simulink model "cochons_nofail"  (R2014b)
settings: Solver=ode45  StartTime=0.0  StopTime=12000  RelTol=1e-3
libraries: simulink x2
settings Model: TunableVars=p  TunableVarsStorageClass=Auto  Creator=ltraonou  LastModifiedBy=ltraonou
settings SolverCC: ShapePreserveControl=EnableAll
settings DataIOCC: FinalStateName=last_state  InitialState=last_state  LimitDataPoints=off  SaveFormat=StructureWithTime  SaveOutput=off  SaveTime=off
settings OptimizationCC: InlineParams=on
settings DebuggingCC: UnderspecifiedInitializationDetection=Classic  MergeDetectMultiDrivingBlocksExec=none  MultiTaskDSMMsg=warning  MultiTaskCondExecSysMsg=none
settings RTWCC: IncludeERTFirstTime=on

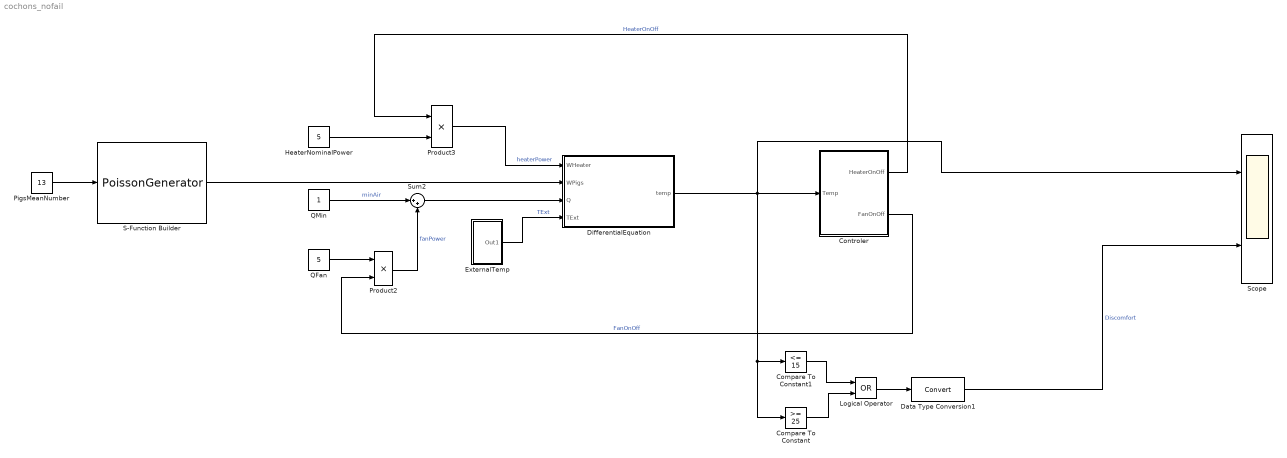
== system cochons_nofail ==
  Compare To Constant : simulink/Logic and Bit Operations/Compare To Constant  relop=>=  const=25  OutDataTypeStr=boolean
  Compare To Constant1 : simulink/Logic and Bit Operations/Compare To Constant  relop=<=  const=15  OutDataTypeStr=boolean
  Controler : Subsystem
  Data Type Conversion1 : DataTypeConversion
  DifferentialEquation : Subsystem
  ExternalTemp : Subsystem
  HeaterNominalPower : Constant  Value=5
  Logical Operator : Logic  Operator=OR  AllPortsSameDT=off  OutDataTypeStr=boolean
  PigsMeanNumber : Constant  Value=13
  Product2 : Product
  Product3 : Product
  QFan : Constant  Value=5
  QMin : Constant
  S-Function Builder : S-Function  InitFcn=try, set_param(gcb,'FunctionName','PoissonGenerator'), end  FunctionName=PoissonGenerator  SFunctionModules=PoissonGenerator_wrapper  EnableBusSupport=off  mask(S-Function Builder){}
      mask help: Simulink:masks:SFunctionBuilder_MD
      mask init:
      | val = [[.9  0.75 0.75 1 1 .9 .9 1]',[1 1 0.75 0.75 .9 .9 1 .9]'];try , sys = get_param(gcb,'SfunBuilderFcnName');if isempty(sys), sys = get_param(gcb,'FunctionName'); end,catch, sys = get_param(gcb,'FunctionName'); end
      settings: CopyFcn=set_param(gcbh,'LinkStatus','none')  PreSaveFcn=try, set_param(gcb,'FunctionName','PoissonGenerator'), end  OpenFcn=sfunctionwizard(gcbh)
      mask Display: plot(val(:,1),val(:,2)),disp(sys), port_label('input',1,'lambda'), port_label('output',1,'y')
  Scope : Scope  NumInputPorts=2
      settings: TimeRange=200000  YMin=-5~-5  YMax=5~5
  Sum2 : Sum  Inputs=|++
  wires:
  QFan/1 -> Product2/1
  QMin/1 -> Sum2/1  "minAir"
  Product2/1 -> Sum2/2  "fanPower"
  Product3/1 -> DifferentialEquation/1(WHeater)  "heaterPower"
  HeaterNominalPower/1 -> Product3/2
  Controler/2(FanOnOff) -> Product2/2  "FanOnOff"
  Controler/1(HeaterOnOff) -> Product3/1  "HeaterOnOff"
  Data Type Conversion1/1 -> Scope/2  "Discomfort"
  DifferentialEquation/1(temp) -> Controler/1(Temp), Scope/1, Compare To Constant/1, Compare To Constant1/1
  S-Function Builder/1 -> DifferentialEquation/2(WPigs)
  Sum2/1 -> DifferentialEquation/3(Q)
  PigsMeanNumber/1 -> S-Function Builder/1
  ExternalTemp/1(Out1) -> DifferentialEquation/4(TExt)  "TExt"
  Compare To Constant1/1 -> Logical Operator/1
  Compare To Constant/1 -> Logical Operator/2
  Logical Operator/1 -> Data Type Conversion1/1

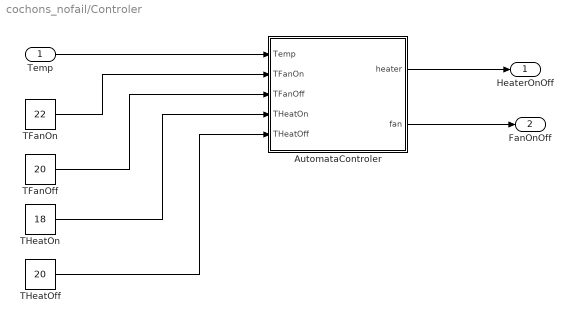
== system cochons_nofail/Controler ==
  Temp : Inport
  AutomataControler : Stateflow chart  TreatAsAtomicUnit=on
  TFanOff : Constant  Value=20
  TFanOn : Constant  Value=22
  THeatOff : Constant  Value=20
  THeatOn : Constant  Value=18
  HeaterOnOff : Outport
  FanOnOff : Outport  Port=2
  wires:
  Temp/1 -> AutomataControler/1(Temp)
  TFanOn/1 -> AutomataControler/2(TFanOn)
  THeatOn/1 -> AutomataControler/4(THeatOn)
  THeatOff/1 -> AutomataControler/5(THeatOff)
  TFanOff/1 -> AutomataControler/3(TFanOff)
  AutomataControler/2(fan) -> FanOnOff/1
  AutomataControler/1(heater) -> HeaterOnOff/1

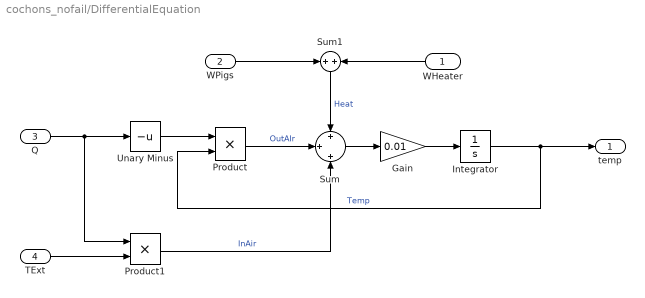
== system cochons_nofail/DifferentialEquation ==
  WHeater : Inport
  WPigs : Inport  Port=2
  Q : Inport  Port=3
  TExt : Inport  Port=4
  Gain : Gain  Gain=0.01
  Integrator : Integrator  InitialCondition=20
  Product : Product
  Product1 : Product
  Sum : Sum  Inputs=+|+|+
  Sum1 : Sum  Inputs=+|+
  Unary Minus : UnaryMinus
  temp : Outport
  wires:
  WHeater/1 -> Sum1/2
  Sum1/1 -> Sum/1  "Heat"
  Unary Minus/1 -> Product/1
  Product1/1 -> Sum/3  "InAir"
  Product/1 -> Sum/2  "OutAIr"
  Q/1 -> Product1/1, Unary Minus/1
  Sum/1 -> Gain/1
  Gain/1 -> Integrator/1
  WPigs/1 -> Sum1/1
  Integrator/1 -> Product/2, temp/1  "Temp"
  TExt/1 -> Product1/2

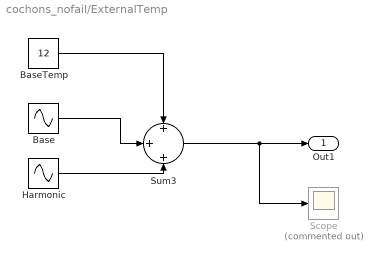
== system cochons_nofail/ExternalTemp ==
  Base : Sin  Amplitude=10  Frequency=0.01  SampleTime=0
  BaseTemp : Constant  Value=12
  Harmonic : Sin  Amplitude=3  Frequency=0.1  SampleTime=0
  Scope : Scope  Commented=on
      settings: TimeRange=11000  SampleInput=on  SampleTime=0.1
  Sum3 : Sum  Inputs=+|+|+
  Out1 : Outport
  wires:
  BaseTemp/1 -> Sum3/1
  Sum3/1 -> Scope/1, Out1/1
  Base/1 -> Sum3/2
  Harmonic/1 -> Sum3/3

== stateflow chart cochons_nofail/Controler/AutomataControler ==
  state Idle
    heater=0;
    fan=0;
  state Fan_on
    heater=0;
    fan=1;
  state Heater_on
    heater=1;
    fan=0;
  (default) -> Idle
  Fan_on -> Idle : [Temp<=TFanOff]
  Idle -> Fan_on [order 1] : [Temp>=TFanOn]
  Idle -> Heater_on [order 2] : [Temp<=THeatOn]
  Heater_on -> Idle : [Temp>=THeatOff]
  data: heater output double; Temp input; fan output double; TFanOn input; TFanOff input; THeatOn input; THeatOff input
